simulink model "NxMultilevelBoostConverterForReport"  (R2018a)
settings: Solver=ode23tb  StartTime=0.0  StopTime=0.3  MaxStep=1e-6  RelTol=1e-3
libraries: powerlib x15, simulink x1
settings Model: Creator=Ilian  LastModifiedBy=Ilian
settings SolverCC: InitialStep=1e-8  ZeroCrossAlgorithm=Adaptive
settings DebuggingCC: MaxConsecutiveZCsMsg=none  MaskedZcDiagnostic=none  IgnoredZcDiagnostic=none  UnconnectedInputMsg=none  UnconnectedOutputMsg=none  UnconnectedLineMsg=none

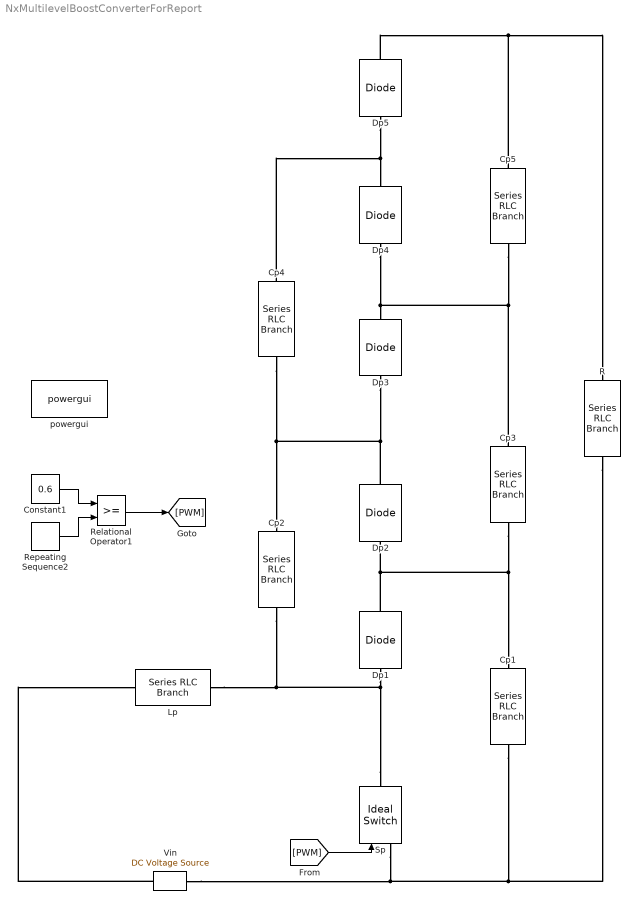
== system NxMultilevelBoostConverterForReport ==
  "\tLp" : powerlib/Elements/Series RLC Branch  LConnTagsString=__new0  RConnTagsString=__new0  BranchType=L  Resistance=1  Inductance=150e-6  SetiL0=off  InitialCurrent=0  Capacitance=1e-6  Setx0=off  InitialVoltage=0  Measurements=Branch voltage and current
  "\tR" : powerlib/Elements/Series RLC Branch  LConnTagsString=__new0  RConnTagsString=__new0  BranchType=R  Resistance=225  Inductance=150e-6  SetiL0=off  InitialCurrent=0  Capacitance=1e-6  Setx0=off  InitialVoltage=0  Measurements=Branch voltage and current
  Constant1 : Constant  Value=0.6
  Cp{1..5} (5 alike) : powerlib/Elements/Series RLC Branch  LConnTagsString=__new0  RConnTagsString=__new0  BranchType=C  Resistance=1  Inductance=150e-3  SetiL0=off  InitialCurrent=0  Capacitance=220e-6  Setx0=off  InitialVoltage=0  Measurements=Branch voltage and current
  Dp{1..5} (5 alike) : powerlib/Power Electronics/Diode  Ron=0.001  Lon=0  Vf=0.8  IC=0  UseSnubber=0  Rs=500  Cs=250e-9  Measurements=off
  Relational Operator1 : RelationalOperator  OutDataTypeStr=boolean  RndMeth=Nearest
  Repeating Sequence2 : simulink/Sources/Repeating Sequence  rep_seq_t=[0 1/50000]  rep_seq_y=[0 1]
  Sp : powerlib/Power Electronics/Ideal Switch  Ron=0.001  Lon=0  IC=0  Rs=1e5  Cs=inf  Measurements=off
  Vin : powerlib/Electrical Sources/DC Voltage Source  Amplitude=10  Measurements=None
  powergui : powerlib/powergui  Priority=1  SimulationMode=Continuous  SampleTime=50e-6  frequency=60  Iterations=50  frequencyindice=0  Pbase=100e6  ErrMax=1e-4  UnitsV=kV  UnitsW=MW  buscounter=0  FunctionMessages=off  echomessages=off  EnableUseOfTLC=off  CurrentSourceSwitches=off  DisableSnubberDevices=off  DisableRonSwitches=off  DisableVfSwitches=off  DisplayEquations=off  SolverType=Tustin/Backward Euler (TBE)  Interpol=off  ExternalGateDelay=off  methode=off  Ts=100  x0status=blocks  SPID=on  SwTol=0  HookPort=off  RestoreLinks=warning  ResistiveCurrentMeasurement=off  Frange=[0:2:500]  Ylog=off  Xlog=on  ShowGrid=off  save=off  variable=ZData  structure=0  ZoomFFT=off  StartTime=0.0  cycles=1  DisplayStyle=1  fundamental=60  FreqAxis=off  MaxFrequency=1000  frequencyindicesteady=1  RmsSteady=1  display=off
  wires:
  Constant1/1 -> Relational Operator1/1
  Repeating Sequence2/1 -> Relational Operator1/2
  Relational Operator1/1 -> [PWM]
  [PWM] -> Sp/1
  connections:
  Vin/RConn1 -- "\tLp"/LConn1
  "\tLp"/RConn1 -- Dp1/LConn1 -- Sp/RConn1 -- Cp2/RConn1
  Sp/LConn1 -- Vin/LConn1 -- "\tR"/RConn1 -- Cp1/RConn1
  Cp3/RConn1 -- Dp1/RConn1 -- Dp2/LConn1 -- Cp1/LConn1
  Dp2/RConn1 -- Cp4/RConn1 -- Cp2/LConn1 -- Dp3/LConn1
  Cp3/LConn1 -- Cp5/RConn1 -- Dp4/LConn1 -- Dp3/RConn1
  Cp4/LConn1 -- Dp5/LConn1 -- Dp4/RConn1
  Dp5/RConn1 -- Cp5/LConn1 -- "\tR"/LConn1
